simulink model "test2"  (R2016a)
settings: Solver=VariableStepAuto  StartTime=0.0  StopTime=10  RelTol=1e-3
settings Model: Creator=mrlisdim  LastModifiedBy=Jann dan Jursus

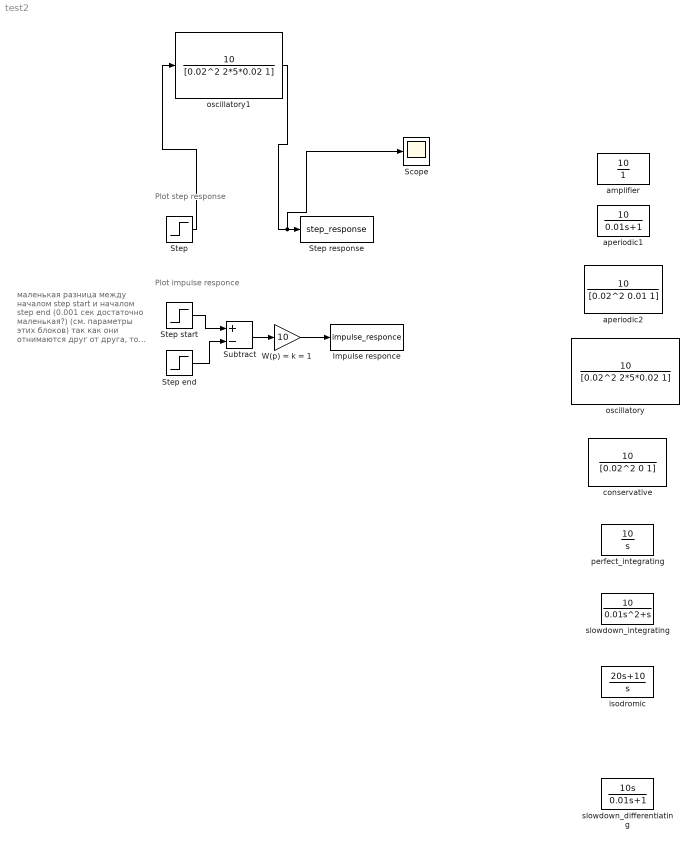
== system test2 ==
  note: маленькая разница
      | между началом step start
      | и началом step end
      | (0.001 сек достаточно
      | маленькая?)
      | (см. параметры этих блоков)
      |
      | так как они отнимаются друг
      | от друга, то получаем типа
      | импульс
  note: Plot impulse responce
  note: Plot step response
  Impulse responce : ToWorkspace  VariableName=impulse_responce  SaveFormat=Timeseries  SampleTime=-1
  Scope : Scope
  Step : Step  Time=0  SampleTime=0
  Step end : Step  Time=1.001  After=100  SampleTime=0
  Step response : ToWorkspace  VariableName=step_response  SaveFormat=Timeseries  SampleTime=-1
  Step start : Step  After=100  SampleTime=0
  Subtract : Sum  Inputs=+-
  W(p) = k = 1 : Gain  Gain=10
  amplifier : TransferFcn  Numerator=[10]  Denominator=[1]
  aperiodic1 : TransferFcn  Numerator=[10]  Denominator=[0.01 1]
  aperiodic2 : TransferFcn  Numerator=[10]  Denominator=[0.02^2 0.01 1]
  conservative : TransferFcn  Numerator=[10]  Denominator=[0.02^2 0 1]
  isodromic : TransferFcn  Numerator=[20 10]  Denominator=[1 0]
  oscillatory : TransferFcn  Numerator=[10]  Denominator=[0.02^2 2*5*0.02 1]
  oscillatory1 : TransferFcn  Numerator=[10]  Denominator=[0.02^2 2*5*0.02 1]
  perfect_integrating : TransferFcn  Numerator=[10]  Denominator=[1 0]
  slowdown_differentiating : TransferFcn  Numerator=[10 0]  Denominator=[0.01 1]
  slowdown_integrating : TransferFcn  Numerator=[10]  Denominator=[0.01 1 0]
  wires:
  Step/1 -> oscillatory1/1
  oscillatory1/1 -> Scope/1, Step response/1
  Step start/1 -> Subtract/1
  Step end/1 -> Subtract/2
  Subtract/1 -> W(p) = k = 1/1
  W(p) = k = 1/1 -> Impulse responce/1
